simulink model "confronto_lineare_non_lineare_osservatore_stato"  (R2018a)
settings: Solver=VariableStepAuto  StartTime=0.0  StopTime=30  RelTol=1e-3
values from neighbouring files (symbols this model uses):
  AO = A - L*C    [osservatore_asintotico.m]
  BO = [B L]    [osservatore_asintotico.m]
  CO = eye(4)    [osservatore_asintotico.m]
  DO = zeros(4,4)    [osservatore_asintotico.m]
  x0 = [0.1,0,0,0]    [main.m]
undefined symbols (not defined in the file or in its folder): A, alpha_eq, B, dati, fd_eq, input, x_eq
settings Model: Creator=Ivonne  LastModifiedBy=Ivonne

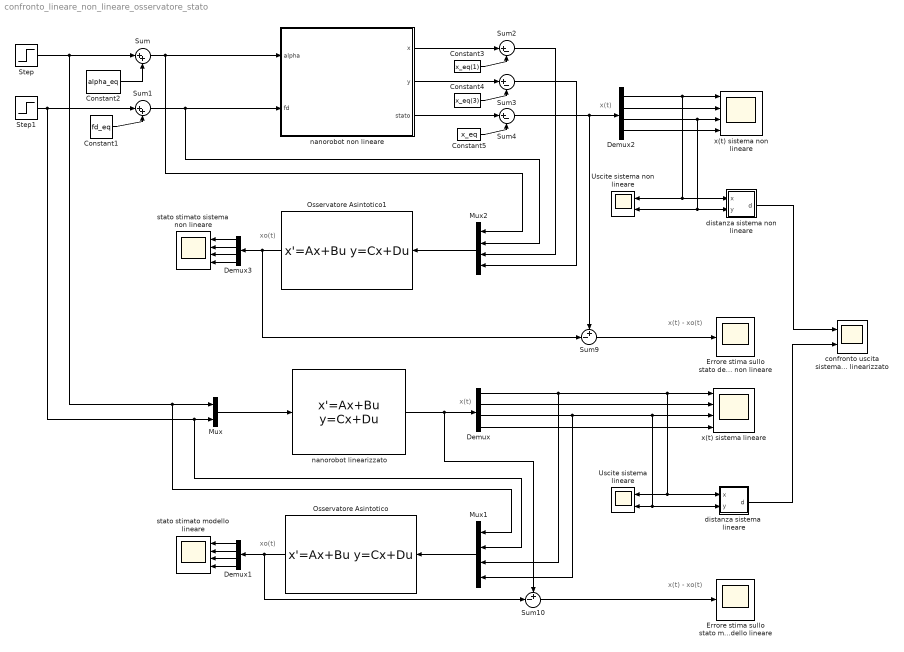
== system confronto_lineare_non_lineare_osservatore_stato ==
  note: x(t)
  note: xo(t)
  note: xo(t)
  note: x(t)
  note: x(t) - xo(t)
  note: x(t) - xo(t)
  Constant1 : Constant  Value=fd_eq
  Constant2 : Constant  Value=alpha_eq
  Constant3 : Constant  Value=x_eq(1)
  Constant4 : Constant  Value=x_eq(3)
  Constant5 : Constant  Value=x_eq
  Demux{,1..3} (4 alike) : Demux
  Errore stima sullo stato del modello non lineare : Scope
  Errore stima sullo stato modello lineare : Scope
  Mux : Mux  Inputs=2
  Mux1 : Mux
  Mux2 : Mux
  Osservatore Asintotico : StateSpace  A=AO  B=BO  C=CO  D=DO  InitialCondition=input
  Osservatore Asintotico1 : StateSpace  A=AO  B=BO  C=CO  D=DO  InitialCondition=input
  Step : Step  SampleTime=0
  Step1 : Step  SampleTime=0
  Sum : Sum  Inputs=|++
  Sum1 : Sum  Inputs=|++
  Sum10 : Sum  Inputs=+-|
  Sum2 : Sum  Inputs=|+-
  Sum3 : Sum  Inputs=|+-
  Sum4 : Sum  Inputs=|+-
  Sum9 : Sum  Inputs=+-|
  Uscite sistema lineare : Scope  NumInputPorts=2
  Uscite sistema non lineare : Scope  NumInputPorts=2
  confronto uscita sistema non lineare e modello linearizzato : Scope  NumInputPorts=2
  "distanza sistema  lineare " : Subsystem
  "distanza sistema non lineare " : Subsystem
  nanorobot linearizzato : StateSpace  A=A  B=B  C=eye(4)  D=zeros(4,2)  InitialCondition=x0
  nanorobot non lineare : Subsystem
  stato stimato sistema non lineare : Scope  NumInputPorts=4
  stato stimato modello lineare : Scope  NumInputPorts=4
  x(t) sistema lineare : Scope  NumInputPorts=4
  x(t) sistema non lineare : Scope  NumInputPorts=4
  wires:
  Constant2/1 -> Sum/2
  Constant1/1 -> Sum1/2
  Mux/1 -> nanorobot linearizzato/1
  nanorobot linearizzato/1 -> Demux/1, Sum10/1
  Constant3/1 -> Sum2/2
  nanorobot non lineare/1(x) -> Sum2/1
  Sum2/1 -> Mux2/3
  nanorobot non lineare/2(y) -> Sum3/1
  Constant4/1 -> Sum3/2
  Sum3/1 -> Mux2/4
  nanorobot non lineare/3(stato) -> Sum4/1
  Constant5/1 -> Sum4/2
  Demux2/4 -> x(t) sistema non lineare/4
  Demux2/1 -> x(t) sistema non lineare/1, "distanza sistema non lineare "/1(x), Uscite sistema non lineare/1
  Demux2/2 -> x(t) sistema non lineare/2
  Demux2/3 -> x(t) sistema non lineare/3, "distanza sistema non lineare "/2(y), Uscite sistema non lineare/2
  Sum/1 -> nanorobot non lineare/1(alpha), Mux2/1
  Sum1/1 -> nanorobot non lineare/2(fd), Mux2/2
  Step/1 -> Mux1/1, Mux/1, Sum/1
  Step1/1 -> Mux1/2, Mux/2, Sum1/1
  Demux/1 -> x(t) sistema lineare/1, "distanza sistema  lineare "/1(x), Uscite sistema lineare/1, Mux1/3
  Demux/3 -> Mux1/4, x(t) sistema lineare/3, Uscite sistema lineare/2, "distanza sistema  lineare "/2(y)
  Demux/2 -> x(t) sistema lineare/2
  Demux/4 -> x(t) sistema lineare/4
  Sum4/1 -> Sum9/1, Demux2/1
  Osservatore Asintotico/1 -> Demux1/1, Sum10/2
  Mux1/1 -> Osservatore Asintotico/1
  Mux2/1 -> Osservatore Asintotico1/1
  Sum9/1 -> Errore stima sullo stato del modello non lineare/1
  Sum10/1 -> Errore stima sullo stato modello lineare/1
  "distanza sistema non lineare "/1(d) -> confronto uscita sistema non lineare e modello linearizzato/1
  "distanza sistema  lineare "/1(d) -> confronto uscita sistema non lineare e modello linearizzato/2
  Osservatore Asintotico1/1 -> Demux3/1, Sum9/2
  Demux1/1 -> stato stimato modello lineare/1
  Demux1/2 -> stato stimato modello lineare/2
  Demux1/3 -> stato stimato modello lineare/3
  Demux1/4 -> stato stimato modello lineare/4
  Demux3/4 -> stato stimato sistema non lineare/4
  Demux3/2 -> stato stimato sistema non lineare/2
  Demux3/1 -> stato stimato sistema non lineare/1
  Demux3/3 -> stato stimato sistema non lineare/3

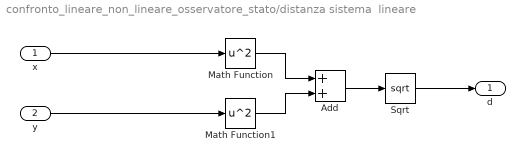
== system confronto_lineare_non_lineare_osservatore_stato/distanza sistema  lineare  ==
  x : Inport
  y : Inport  Port=2
  Add : Sum
  Math Function : Math  Operator=square  SaturateOnIntegerOverflow=on
  Math Function1 : Math  Operator=square  SaturateOnIntegerOverflow=on
  Sqrt : Sqrt  SaturateOnIntegerOverflow=on
  d : Outport
  wires:
  Add/1 -> Sqrt/1
  x/1 -> Math Function/1
  Math Function/1 -> Add/1
  Math Function1/1 -> Add/2
  Sqrt/1 -> d/1
  y/1 -> Math Function1/1

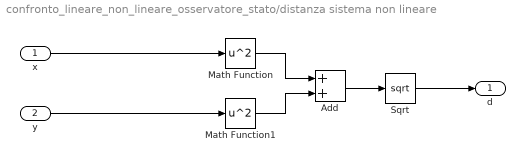
== system confronto_lineare_non_lineare_osservatore_stato/distanza sistema non lineare  ==
  x : Inport
  y : Inport  Port=2
  Add : Sum
  Math Function : Math  Operator=square  SaturateOnIntegerOverflow=on
  Math Function1 : Math  Operator=square  SaturateOnIntegerOverflow=on
  Sqrt : Sqrt  SaturateOnIntegerOverflow=on
  d : Outport
  wires:
  Add/1 -> Sqrt/1
  x/1 -> Math Function/1
  Math Function/1 -> Add/1
  Math Function1/1 -> Add/2
  Sqrt/1 -> d/1
  y/1 -> Math Function1/1

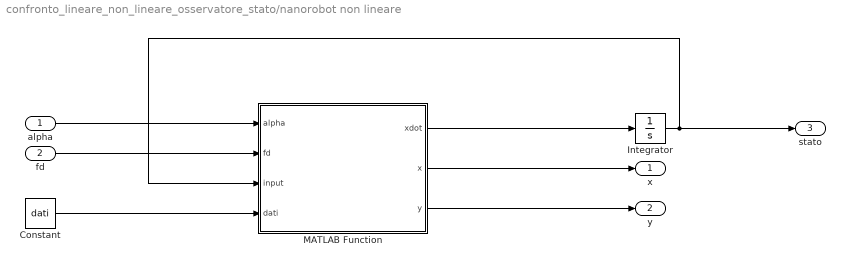
== system confronto_lineare_non_lineare_osservatore_stato/nanorobot non lineare ==
  alpha : Inport
  fd : Inport  Port=2
  Constant : Constant  Value=dati
  Integrator : Integrator  InitialCondition=x0
  MATLAB Function : MATLAB Function  TreatAsAtomicUnit=on
  x : Outport
  y : Outport  Port=2
  stato : Outport  Port=3
  wires:
  MATLAB Function/1(xdot) -> Integrator/1
  Integrator/1 -> stato/1, MATLAB Function/3(input)
  MATLAB Function/2(x) -> x/1
  Constant/1 -> MATLAB Function/4(dati)
  alpha/1 -> MATLAB Function/1(alpha)
  MATLAB Function/3(y) -> y/1
  fd/1 -> MATLAB Function/2(fd)

== matlab function confronto_lineare_non_lineare_osservatore_stato/nanorobot non lineare/MATLAB Function ==
  data: xdot output; alpha input; fd input; input input; x output; dati input; y output
function [ xdot, x, y ] = fcn(alpha, fd, input, dati)
% input : condizioni iniziali
% u : ingresso del sistema -> [ alpha, fd]
% dati : parametri del modello fisico -> [ R, Fm, m, eta,l, dP, r, vf ]
R= dati(1);                 
Fm = dati(2);  
m = dati(3);
eta = dati(4);
l = dati(5);
dP = dati(6);
r = dati(7);
vf = dati(8);
% variabili di stato 
% x1 = x, x2 = xp -> x1p, x3 = y, x4 = yp -> x3p
% allora xpp = x2p e ypp = x4p
x1 = input(1); % xdot(1) = x2 -> 1/s 
x2 = input(2); % xdot(2) = x2p -> 1/s 
x3 = input(3); % xdot(3) = x4 -> 1/s
x4 = input(4); % xdot(4) = x4p -> 1/s
% forma di stato
xdot = [ x2;
         ((-6*pi*eta*R)/m)*x2 + ((6*pi*eta*R)/m)*vf + (Fm/m)*cos(alpha) + fd/m;
         x4;
         ((-6*pi*eta*R)/m)*x4 + (Fm/m)*sin(alpha)];

% coordinate cartesiane
x = x1;
y = x3;
